simulink model "freq_support_qpoases"  (R2022a)
settings: Solver=VariableStepAuto  StartTime=0.0  StopTime=50  FixedStep=0.02  MaxStep=1e-3  RelTol=1e-3
InitFcn:
  | M = 4; D = 1.5/100; Rp = 0.05; Tg = 0.2; Ki = 1.8;
libraries: commchan3 x1
settings Model: Creator=Niranjan.Bhujel  LastModifiedBy=niran
settings SolverCC: AlgebraicLoopSolver=TrustRegion
settings DebuggingCC: UnconnectedInputMsg=warning  UnconnectedOutputMsg=warning  UnconnectedLineMsg=warning  SFMachineParentedDataDiag=warning

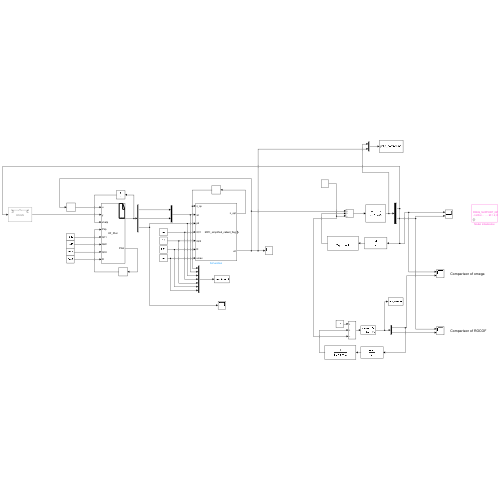
[thumbnail: Simulink's stored preview of the top-level diagram]
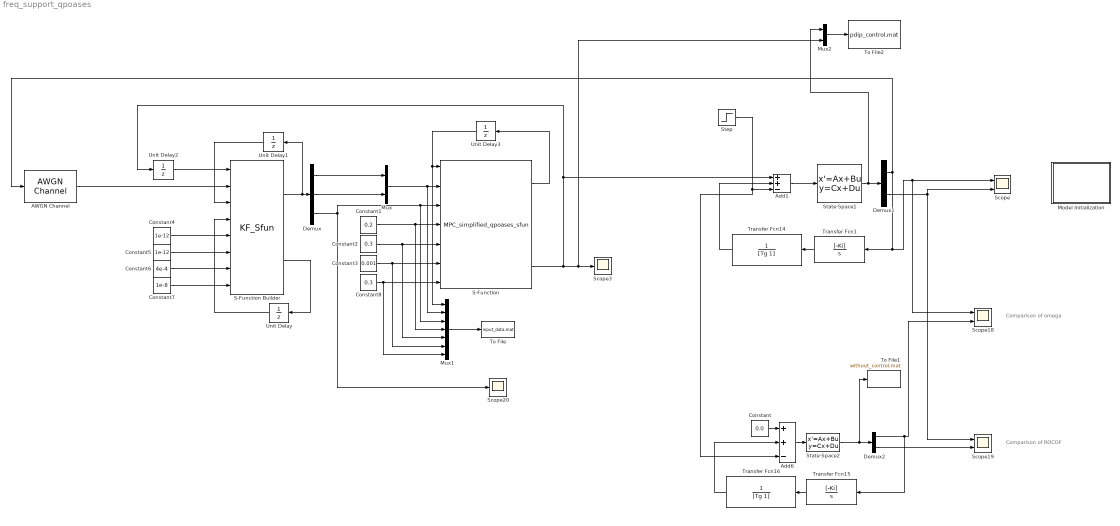
== system freq_support_qpoases ==
  note: Comparison of omega
  note: Comparison of ROCOF
  AWGN Channel : commchan3/AWGN Channel  InputProcessing=Columns as channels (frame based)  seed=67  noiseMode=Variance from mask  EbNodB=10  EsNodB=10  SNRdB=10  bitsPerSym=1  Ps=1  Tsym=1  variance=1e-11
  Add1 : Sum  Inputs=++-
  Add6 : Sum  Inputs=++-
  Constant : Constant  Value=0.0
  Constant1 : Constant  Value=0.2
  Constant2 : Constant  Value=0.3
  Constant3 : Constant  Value=0.001
  Constant4 : Constant  Value=1e-12
  Constant5 : Constant  Value=1e-12
  Constant6 : Constant  Value=4e-4
  Constant7 : Constant  Value=1e-8
  Constant8 : Constant  Value=0.3
  Demux : Demux  Outputs=3
  Demux1 : Demux  Outputs=2
  Demux2 : Demux  Outputs=2
  Model Initialization : Subsystem  mask(Model Functions){InitFcnX=M = 4; D = 1.5/100; Rp = 0.05; Tg = 0.2; Ki = 1.8;, prel=off, posl=off, inif=on, strf=off}
      mask prompts: InitFcnX "Initialisation"; prel "Preload Function"; posl "PostLoad Function"; inif "InitFcn"; strf "StartFcn"
      mask init:
      | currentBlock = gcb;
      | root = bdroot(currentBlock);
      | 
      | if ~strcmp(get_param(root,'BlockDiagramType'),'library')
      |     if prel==1
      |         set_param(root, 'PreLoadFcn', InitFcnX);
      |     else
      |         set_param(root, 'PreLoadFcn', '');
      |     end
      |     if inif==1
      |         set_param(root, 'InitFcn', InitFcnX);
      |     else
      |         set_param(root, 'InitFcn', '');
      |     end
      |     if strf==1
      |         set_param(root, 'StartFcn', InitFcnX);
      |     else
      |         set_param(root, 'StartFcn', '');
      |     end
      |     if posl==1
      |         set_param(root, 'PostLoadFcn', InitFcnX);
      |     else
      |         set_param(root, 'PostLoadFcn', '');
      |     end
      | end
      | 
      | pos = get_param(currentBlock, 'Position');
      | width = pos(3) - pos(1); height = pos(4) - pos(2);
      | txt = [ upper(root) '\n' '- InitFcn. . . . . '  get_param(root, 'InitFcn') ];
      settings: CopyFcn=set_param(gcb,'LinkStatus','inactive')
      mask Display: text(5, height*0.5, txt, 'horizontalAlignment', 'left', 'verticalAlignment', 'middle') ;
  Mux : Mux  Inputs=2
  Mux1 : Mux  Inputs=7
  Mux2 : Mux  Inputs=2
  S-Function : S-Function  FunctionName=MPC_simplified_qpoases_sfun  SFunctionDeploymentMode=off  EnableBusSupport=off
      mask Display:
      | %% S-Function mask command
      | port_label('input', 1, 'z_op');
      | port_label('input', 2, 'x0');
      | port_label('input', 3, 'pd');
      | port_label('input', 4, 'Q11');
      | port_label('input', 5, 'Q22');
      | port_label('input', 6, 'R');
      | port_label('input', 7, 'umax');
      | port_label('output', 1, 'z_opt');
      | port_label('output', 2, 'exit_flag');
      | port_label('output', 3, 'u0');
      | disp('MPC_simplified_call');
  S-Function Builder : S-Function  InitFcn=try, set_param(gcb,'FunctionName','KF_Sfun'), end  FunctionName=KF_Sfun  SFunctionModules=KF_Sfun_wrapper EKF_Func EKF_Func_Call  SFunctionDeploymentMode=off  EnableBusSupport=off  mask(S-Function Builder){}
      mask help: Simulink:masks:SFunctionBuilder_MD
      mask init:
      | val = [[.9  0.75 0.75 1 1 .9 .9 1]',[1 1 0.75 0.75 .9 .9 1 .9]'];try , sys = get_param(gcb,'SfunBuilderFcnName');if isempty(sys), sys = get_param(gcb,'FunctionName'); end,catch, sys = get_param(gcb,'FunctionName'); end
      settings: CopyFcn=set_param(gcbh,'LinkStatus','none')  PreSaveFcn=try, set_param(gcb,'FunctionName','KF_Sfun'), end  OpenFcn=sfunctionwizard(gcbh)
      mask Display:
      | plot(val(:,1),val(:,2))
      | disp(sys)
      | port_label('input',1,'u')
      | port_label('input',2,'y')
      | port_label('input',3,'xhatp')
      | port_label('input',4,'Pkp')
      | port_label('input',5,'Q11')
      | port_label('input',6,'Q22')
      | port_label('input',7,'Q33')
      | port_label('input',8,'R')
      | port_label('output',1,'xhat')
      | port_label('output',2,'Phat')
  Scope : Scope  NumInputPorts=2
  Scope18 : Scope  NumInputPorts=2
  Scope19 : Scope  NumInputPorts=2
  Scope20 : Scope
  Scope3 : Scope
  State-Space1 : StateSpace  A=[0 1;-(D/(M*Tg)+1/(Rp*M*Tg)) -(D/M + 1/Tg)]  B=[0;1/(M*Tg)]  C=eye(2)  D=zeros(2,1)  InitialCondition=0
  State-Space2 : StateSpace  A=[0 1;-(D/(M*Tg)+1/(Rp*M*Tg)) -(D/M + 1/Tg)]  B=[0;1/(M*Tg)]  C=eye(2)  D=zeros(2,1)  InitialCondition=0
  Step : Step  Time=10  After=0.75  SampleTime=0
  To File : ToFile  Filename=input_data.mat  SampleTime=0.02
  To File1 : ToFile  Filename=without_control.mat  MatrixName=datavar  SampleTime=0.02
  To File2 : ToFile  Filename=pdip_control.mat  MatrixName=datavar  SampleTime=0.02
  Transfer Fcn1 : TransferFcn  Numerator=[-Ki]  Denominator=[1 0]
  Transfer Fcn14 : TransferFcn  Denominator=[Tg 1]
  Transfer Fcn15 : TransferFcn  Numerator=[-Ki]  Denominator=[1 0]
  Transfer Fcn16 : TransferFcn  Denominator=[Tg 1]
  Unit Delay : UnitDelay  InitialCondition=1*diag([1, 1, 1])  SampleTime=0.02  HasFrameUpgradeWarning=on
  Unit Delay1 : UnitDelay  SampleTime=0.02  HasFrameUpgradeWarning=on
  Unit Delay2 : UnitDelay  SampleTime=0.02  HasFrameUpgradeWarning=on
  Unit Delay3 : UnitDelay  SampleTime=0.02  HasFrameUpgradeWarning=on
  wires:
  Step/1 -> Add6/3, Add1/3
  Add1/1 -> State-Space1/1
  State-Space1/1 -> Mux2/1, Demux1/1
  Transfer Fcn1/1 -> Transfer Fcn14/1
  Demux1/1 -> AWGN Channel/1, Transfer Fcn1/1, Scope18/1, Scope/1
  Demux1/2 -> Scope19/1, Scope/2
  Transfer Fcn15/1 -> Transfer Fcn16/1
  Add6/1 -> State-Space2/1
  Transfer Fcn16/1 -> Add6/2
  State-Space2/1 -> To File1/1, Demux2/1
  Demux2/1 -> Transfer Fcn15/1, Scope18/2
  Transfer Fcn14/1 -> Add1/2
  Demux2/2 -> Scope19/2
  S-Function/3 -> Mux2/2, Scope3/1, Unit Delay2/1, Add1/1
  Constant/1 -> Add6/1
  Constant1/1 -> Mux1/4, S-Function/4
  Constant2/1 -> Mux1/5, S-Function/5
  Constant3/1 -> Mux1/6, S-Function/6
  Demux/3 -> Scope20/1, Mux1/3, S-Function/3
  S-Function Builder/1 -> Unit Delay1/1, Demux/1
  S-Function Builder/2 -> Unit Delay/1
  Unit Delay/1 -> S-Function Builder/4
  Unit Delay1/1 -> S-Function Builder/3
  Unit Delay2/1 -> S-Function Builder/1
  Constant4/1 -> S-Function Builder/5
  Constant5/1 -> S-Function Builder/6
  Constant6/1 -> S-Function Builder/7
  Constant7/1 -> S-Function Builder/8
  AWGN Channel/1 -> S-Function Builder/2
  S-Function/1 -> Unit Delay3/1
  Unit Delay3/1 -> Mux1/1, S-Function/1
  Mux/1 -> Mux1/2, S-Function/2
  Constant8/1 -> Mux1/7, S-Function/7
  Mux1/1 -> To File/1
  Demux/2 -> Mux/2
  Demux/1 -> Mux/1
  Mux2/1 -> To File2/1

== system freq_support_qpoases/Model Initialization ==
